simulink library "Aero_Lib"  (Simulink 8.4)
settings: Solver=ode45  StartTime=0.0  StopTime=10.0  RelTol=1e-3
values from neighbouring files (symbols this model uses):
  AC = miniMUTT_rigid_config    [UAV_config.m]    (also in UAV_modelconfig.mat = )
libraries: UltraStick120_Aero_Lib x2, miniMUTT_rigid_Aero_Lib x2, Aero_Lib x1, simulink x1, UltraStick25e_Aero_Lib x1, aerolibadyn x1
settings Model: ForwardingTableString=||__slOldName__||Aero_Lib/old miniMUTT||__slNewName__||old_miniMUTT_Lib/rigid miniMUTT  Creator=austinmurch  LastModifiedBy=pseiler

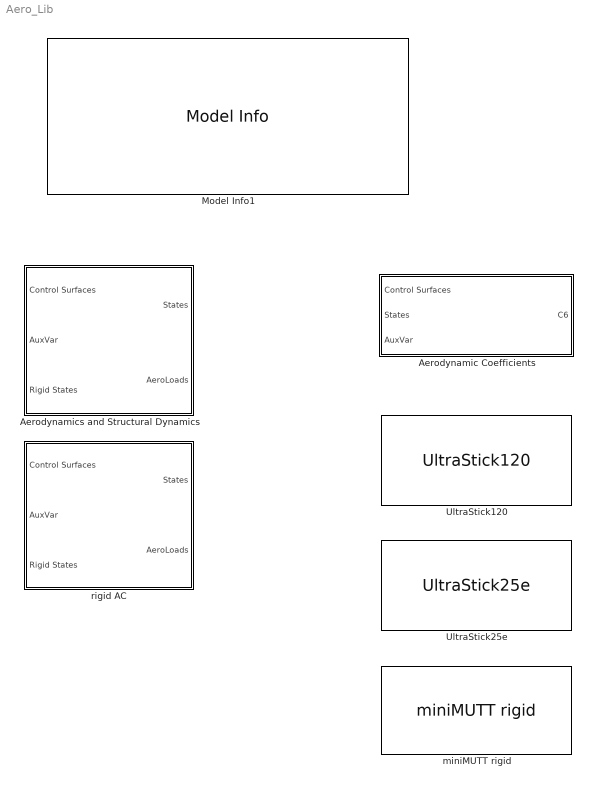
== system Aero_Lib ==
  Aerodynamic Coefficients : Subsystem  BlockChoice=UltraStick120
      settings: TemplateBlock=self  MemberBlocks=UltraStick120,UltraStick25e,miniMUTT rigid,rigid miniMUTT
  Aerodynamics and Structural Dynamics : Subsystem  BlockChoice=rigid AC  mask{aircraft=AC.aircraft}
      mask prompts: aircraft "Aircraft model:"
      mask help: Select aerodynamic model based on AC.aircraft variable
      mask init:
      | pathname = gcb;
      | 
      | switch lower(aircraft)
      |     case 'ultrastick120'
      |         set_param(pathname,'BlockChoice','rigid AC');
      |         set_param([pathname '/rigid AC/Aerodynamic Coefficients'],'BlockChoice','UltraStick120');
      | %         set_param([pathname '/UltraStick/Forces and Moments Calculation'],'inputAxes','Stability');
      | %         set_param([pathname '/UltraStick/Forces and Moments Calculation'],'outputMomentAxes','Stability');
      |     case 'ultrastick25e'
      |         set_param(pathname,'BlockChoice','rigid AC');
      |         set_param([pathname '/rigid AC/Aerodynamic Coefficients'],'BlockChoice','UltraStick25e');
      | %         set_param([pathname '/UltraStick/Forces and Moments Calculation'],'inputAxes','Wind');
      | %         set_param([pathname '/UltraStick/Forces and Moments Calculation'],'outputMomentAxes','Wind');
      |     case 'minimutt_rigid'
      |     %% Choose these two lines to select the minimutt model
      |     %% with aerodynamic coeffcients
      |         set_param(pathname,'BlockChoice','rigid AC');
      |         set_param([pathname '/rigid AC/Aerodynamic Coefficients'],'BlockChoice','miniMUTT rigid');
      | end
      settings: TemplateBlock=self  MemberBlocks=rigid AC
  Model Info1 : simulink/Model-Wide Utilities/Model Info  BlockCM=None  Frame=on  DisplayStringWithTags=|  HorizontalTextAlignment=Left  LeftAlignmentValue=0.02  SourceBlockDiagram=Aero_Lib  TagMaxNumber=20
      | MODEL INFORMATION
      | Aerodynamic Model Library
      | 
      | University of Minnesota
      | Aerospace Engineering and Mechanics
      | Copyright 2011 Regents of the University of Minnesota. All rights reserved.
      | 
      | == SVN Info ==
      | Last modified by %<LastModifiedBy> on %<LastModificationDate>
  UltraStick120 : UltraStick120_Aero_Lib/UltraStick120
  UltraStick25e : UltraStick25e_Aero_Lib/UltraStick25e
  miniMUTT rigid : miniMUTT_rigid_Aero_Lib/miniMUTT rigid
  rigid AC : Subsystem  mask{aircraft=AC.aircraft}
      mask prompts: aircraft "Aircraft Type:"
      mask init:
      | pathname = gcb;
      | 
      | switch lower(aircraft)
      |     case 'ultrastick120'
      |         set_param([pathname '/Forces and Moments Calculation'],'inputAxes','Stability');
      |         set_param([pathname '/Forces and Moments Calculation'],'outputMomentAxes','Stability');
      |     case 'ultrastick25e'
      |         set_param([pathname '/Forces and Moments Calculation'],'inputAxes','Wind');
      |         set_param([pathname '/Forces and Moments Calculation'],'outputMomentAxes','Wind');
      |     case 'minimutt_rigid'
      |         set_param([pathname '/Forces and Moments Calculation'],'inputAxes','Wind');
      |         set_param([pathname '/Forces and Moments Calculation'],'outputForceAxes','Wind');        
      |         set_param([pathname '/Forces and Moments Calculation'],'outputMomentAxes','Wind');        
      | end

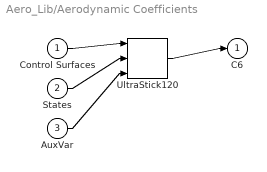
== system Aero_Lib/Aerodynamic Coefficients ==
  Control Surfaces : Inport
  States : Inport  Port=2
  AuxVar : Inport  Port=3
  UltraStick120 : UltraStick120_Aero_Lib/UltraStick120
  C6 : Outport
  wires:
  Control Surfaces/1 -> UltraStick120/1
  States/1 -> UltraStick120/2
  AuxVar/1 -> UltraStick120/3
  UltraStick120/1 -> C6/1

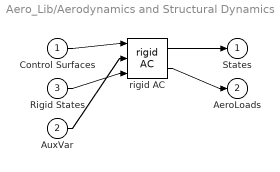
== system Aero_Lib/Aerodynamics and Structural Dynamics ==
  Control Surfaces : Inport
  AuxVar : Inport  Port=2
  Rigid States : Inport  Port=3
  rigid AC : Aero_Lib/rigid AC  aircraft=AC.aircraft
      link override Aerodynamic Coefficients: BlockChoice=rigid miniMUTT
  States : Outport
  AeroLoads : Outport  Port=2
  wires:
  Control Surfaces/1 -> rigid AC/1
  AuxVar/1 -> rigid AC/2
  Rigid States/1 -> rigid AC/3
  rigid AC/1 -> States/1
  rigid AC/2 -> AeroLoads/1

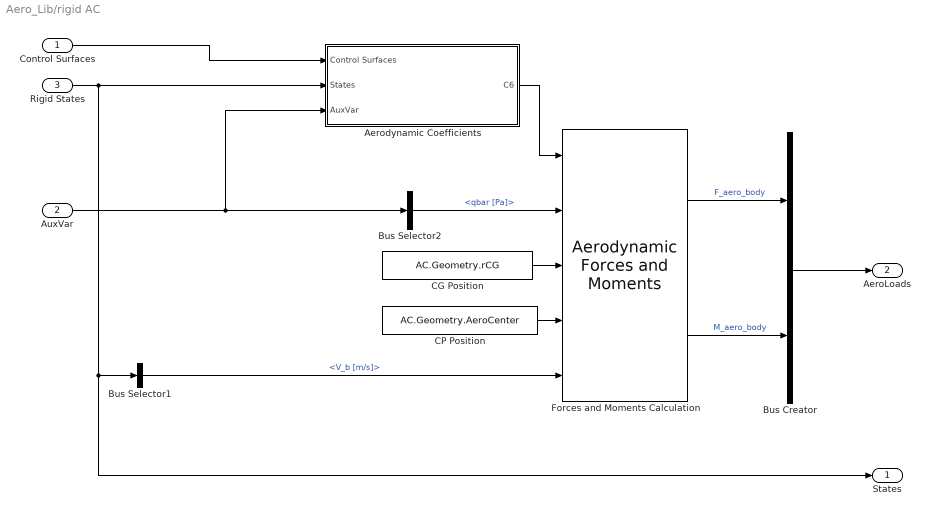
== system Aero_Lib/rigid AC ==
  Control Surfaces : Inport
  AuxVar : Inport  Port=2
  Rigid States : Inport  Port=3
  Aerodynamic Coefficients : Subsystem  BlockChoice=miniMUTT rigid
      settings: AttributesFormatString=%<BlockChoice>  TemplateBlock=Aero_Lib/Aerodynamic Coefficients  MemberBlocks=UltraStick120,UltraStick25e,miniMUTT rigid,rigid miniMUTT
  Bus Selector1 : BusSelector  OutputSignals=V_b [m/s]
  Bus Creator : BusCreator  Inputs=2
  Bus Selector2 : BusSelector  OutputSignals=qbar [Pa]
  CG Position : Constant  Value=AC.Geometry.rCG
  CP Position : Constant  Value=AC.Geometry.AeroCenter
  Forces and Moments Calculation : aerolibadyn/Aerodynamic Forces and Moments   inputAxes=Wind  outputForceAxes=Wind  outputMomentAxes=Wind  S=AC.Geometry.S  b=AC.Geometry.b  cbar=AC.Geometry.c
  States : Outport
  AeroLoads : Outport  Port=2
  wires:
  Bus Selector1/1 -> Forces and Moments Calculation/5  "<V_b [m/s]>"
  CG Position/1 -> Forces and Moments Calculation/3
  CP Position/1 -> Forces and Moments Calculation/4
  Rigid States/1 -> Aerodynamic Coefficients/2(States), States/1, Bus Selector1/1
  Forces and Moments Calculation/1 -> Bus Creator/1  "F_aero_body"
  Bus Creator/1 -> AeroLoads/1
  Forces and Moments Calculation/2 -> Bus Creator/2  "M_aero_body"
  AuxVar/1 -> Aerodynamic Coefficients/3(AuxVar), Bus Selector2/1
  Bus Selector2/1 -> Forces and Moments Calculation/2  "<qbar [Pa]>"
  Aerodynamic Coefficients/1(C6) -> Forces and Moments Calculation/1
  Control Surfaces/1 -> Aerodynamic Coefficients/1(Control Surfaces)

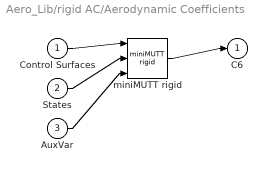
== system Aero_Lib/rigid AC/Aerodynamic Coefficients ==
  Control Surfaces : Inport
  States : Inport  Port=2
  AuxVar : Inport  Port=3
  miniMUTT rigid : miniMUTT_rigid_Aero_Lib/miniMUTT rigid
  C6 : Outport
  wires:
  Control Surfaces/1 -> miniMUTT rigid/1
  States/1 -> miniMUTT rigid/2
  AuxVar/1 -> miniMUTT rigid/3
  miniMUTT rigid/1 -> C6/1
